simulink model "SMO_atan2_disc_model"  (R2024b)
settings: Solver=ode23  StartTime=0.0  StopTime=0.2  FixedStep=2e-7  RelTol=1e-3
InitFcn:
  | pn = 4;
  | Ld = 8.5e-3;
  | Lq = 8.5e-3;
  | Ls = Ld;
  | R = 2.875;
  | phi = 0.175;
  | J = 0.001;
  | B = 0.000;
undefined symbols (not defined in the file or in its folder): DiscIntNeverNeededParam
libraries: spsGroundLib x1, spsUniversalBridgeLib x1, spsPermanentMagnetSynchronousMachineLib x1, spsSVPWMGenerator2LevelLib x1, spsThreePhaseVIMeasurementLib x1, spsDCVoltageSourceLib x1, sps_lib x1

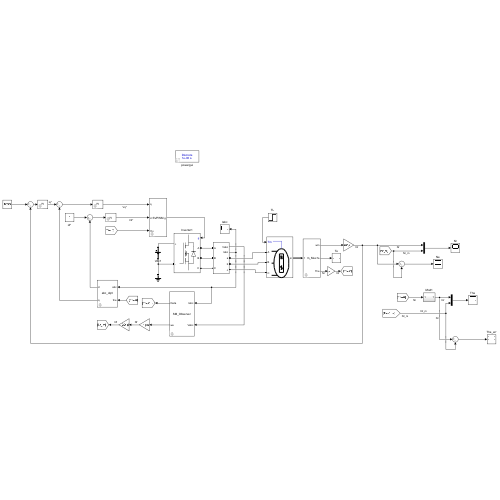
[thumbnail: Simulink's stored preview of the top-level diagram]
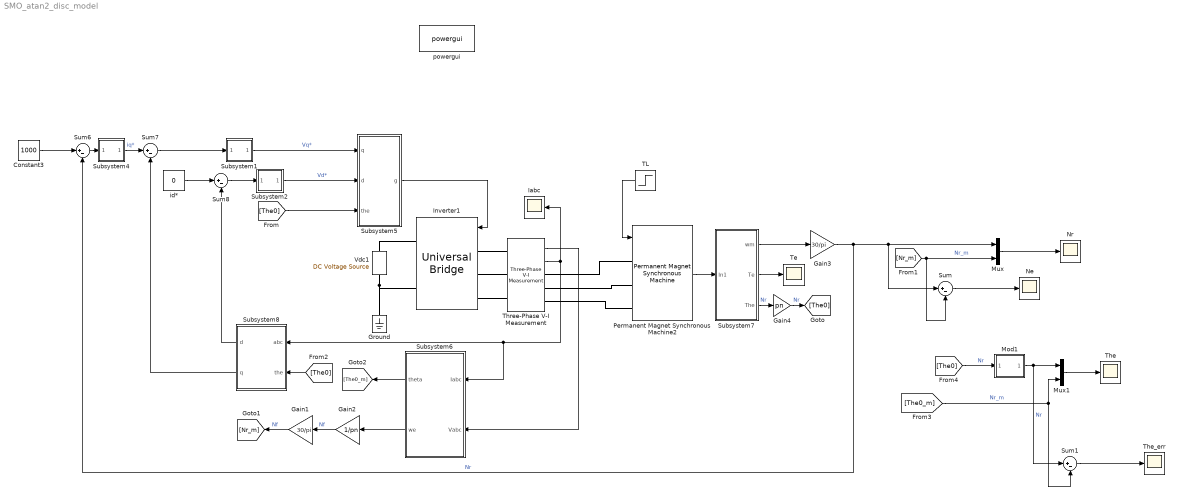
== system SMO_atan2_disc_model ==
  Constant3 : Constant  Value=1000
  Gain1 : Gain  Gain=30/pi
  Gain2 : Gain  Gain=1/pn
  Gain3 : Gain  Gain=30/pi
  Gain4 : Gain  Gain=pn
  Ground : spsGroundLib/Ground  LConnTagsString=a
  Iabc : Scope
  Inverter1 : spsUniversalBridgeLib/Universal Bridge  Arms=3  SnubberResistance=1e5  SnubberCapacitance=inf  Device=MOSFET / Diodes  Ron=1e-3  Lon=0  ForwardVoltages="[  0  0  ]"  ForwardVoltage=0  GTOparameters=[ 10e-6 , 20e-6 ]  IGBTparameters=[ 1e-6 , 2e-6 ]  Measurements=None  Measurements_2=None  converterType=Rectifier
  Mod1 : Subsystem
  Mux : Mux  Inputs=2
  Mux1 : Mux  Inputs=2
  Ne : Scope
  Nr : Scope
  Permanent Magnet Synchronous Machine2 : spsPermanentMagnetSynchronousMachineLib/Permanent Magnet Synchronous Machine  NbPhases=3  FluxDistribution=Sinusoidal  RotorType=Salient-pole  MechanicalLoad=Torque Tm  PresetModel=No  ShowDetailedParameters=on  MeasurementBus=off  Resistance=R  Inductance=8.5e-3  dqInductances=[Ld Lq]  La=0.000395  MachineConstant=Flux linkage established by magnets (V.s)  Flux=0.175  VoltageCst=126.966  TorqueCst=1.05  Flat=120  Mechanical=[J B pn 0]  PolePairs=2  InitialConditions=[0,0, 0,0]  InitialConditions5ph=[0 0 0 0 0 0]  RefAngle=Aligned with phase A axis (original Park)  IterativeDiscreteModel=Trapezoidal non iterative  TsBlock=-1  TsPowergui=0
  Subsystem1 : Subsystem  mask{Ki=2000*R, Kp=2000*Lq, int_limit=[-161,161], out_limit=[-161,161], Ts=1/(10e3)}
      mask prompts: Ki "Ki : Integral"; Kp "Kp : Propotional"; int_limit "integral limit : [min, max]"; out_limit "output limit : [min, max]"; Ts "Ts : sample time"
  Subsystem2 : Subsystem  mask{Ki=2000*R, Kp=2000*Ld, int_limit=[-161,161], out_limit=[-161,161], Ts=1/(10e3)}
      mask prompts: Ki "Ki : Integral"; Kp "Kp : Propotional"; int_limit "integral limit : [min, max]"; out_limit "output limit : [min, max]"; Ts "Ts : sample time"
  Subsystem4 : Subsystem  mask{Ki=25, Kp=0.15, int_limit=[-21,21], out_limit=[-21,21], Ts=1/(5e3)}
      mask prompts: Ki "Ki : Integral"; Kp "Kp : Propotional"; int_limit "integral limit : [min, max]"; out_limit "output limit : [min, max]"; Ts "Ts : sample time"
  Subsystem5 : Subsystem  mask{Vdc=311}
  Subsystem6 : Subsystem  mask{Ts=1/(10e3), wc=5}
      mask prompts: Ts "Ts : sample time"; wc "wc : cross frequency (rad/s)"
  Subsystem7 : Subsystem
  Subsystem8 : Subsystem
  Sum{,1,6..8} (5 alike) : Sum  Inputs=|+-
  TL : Step  Time=0.1  After=10  SampleTime=0
  Te : Scope
  The : Scope
  The_err : Scope
  Three-Phase V-I Measurement : spsThreePhaseVIMeasurementLib/Three-Phase V-I Measurement  VoltageMeasurement=phase-to-ground  SetLabelV=off  LabelV=Vabc  Vpu=off  VpuLL=off  CurrentMeasurement=yes  SetLabelI=off  LabelI=Iabc  Ipu=off  Pbase=100e6  Vbase=500e3  OutputType=Complex  PhasorSimulation=off  PSBequivalent=0
  Vdc1 : spsDCVoltageSourceLib/DC Voltage Source  Amplitude=311  Measurements=None
  id* : Constant  Value=0
  powergui : sps_lib/powergui  Priority=1  SimulationMode=Discrete  SampleTime=10e-7  frequency=60  Iterations=50  frequencyindice=0  Pbase=100e6  ErrMax=1e-4  UnitsV=kV  UnitsW=MW  buscounter=0  FunctionMessages=off  echomessages=off  EnableUseOfTLC=off  CurrentSourceSwitches=off  DisableSnubberDevices=off  DisableRonSwitches=off  DisableVfSwitches=off  DisplayEquations=off  AutomaticDiscreteSolvers=off  SolverType=Tustin/Backward Euler (TBE)  Interpol=off  ExternalGateDelay=off  methode=off  Ts=100  x0status=blocks  SPID=on  SwTol=0  HookPort=off  NonlinearTolerance=1e-4  nMaxIteration=100  ContinueOnMaxIteration=off  RestoreLinks=warning  ResistiveCurrentMeasurement=off  Frange=[0:2:500]  Ylog=off  Xlog=on  ShowGrid=off  save=off  variable=ZData  structure=0  ZoomFFT=off  StartTime=0.0  cycles=1  DisplayStyle=1  fundamental=60  FreqAxis=off  MaxFrequency=1000  frequencyindicesteady=1  RmsSteady=1  display=off
  wires:
  Three-Phase V-I Measurement/2 -> Subsystem8/1(abc), Subsystem6/1(Iabc), Iabc/1
  Sum7/1 -> Subsystem1/1(Input)
  Sum6/1 -> Subsystem4/1(Input)
  Three-Phase V-I Measurement/1 -> Subsystem6/2(Vabc)
  Subsystem4/1(output) -> Sum7/1  "iq*"
  Constant3/1 -> Sum6/1
  Subsystem5/1(g) -> Inverter1/1
  Subsystem7/1(wm) -> Gain3/1
  id*/1 -> Sum8/1
  Subsystem1/1(output) -> Subsystem5/1(q)  "Vq*"
  Sum8/1 -> Subsystem2/1(Input)
  Subsystem2/1(output) -> Subsystem5/2(d)  "Vd*"
  Subsystem8/1(d) -> Sum8/2
  Subsystem8/2(q) -> Sum7/2
  Subsystem7/2(Te) -> Te/1
  [The0] -> Subsystem5/3(the)
  Gain2/1 -> Gain1/1  "Nf"
  Subsystem6/2(we) -> Gain2/1
  Gain3/1 -> Sum6/2, Mux/1, Sum/1  "Nr"
  Mux/1 -> Nr/1
  Sum/1 -> Ne/1
  Subsystem7/3(The) -> Gain4/1  "Nr"
  TL/1 -> Permanent Magnet Synchronous Machine2/1
  Permanent Magnet Synchronous Machine2/1 -> Subsystem7/1(In1)
  [The0] -> Subsystem8/2(the)
  Gain4/1 -> [The0]  "Nr"
  Gain1/1 -> [Nr_m]  "Nf"
  [Nr_m] -> Sum/2, Mux/2  "Nr_m"
  Subsystem6/1(theta) -> [The0_m]
  [The0] -> Mod1/1(In1)  "Nr"
  Mux1/1 -> The/1
  [The0_m] -> Mux1/2, Sum1/2  "Nr_m"
  Mod1/1(Out1) -> Sum1/1, Mux1/1  "Nr"
  Sum1/1 -> The_err/1
  connections:
  Vdc1/LConn1 -- Inverter1/RConn2 -- Ground/LConn1
  Three-Phase V-I Measurement/LConn3 -- Inverter1/LConn3
  Vdc1/RConn1 -- Inverter1/RConn1
  Three-Phase V-I Measurement/LConn2 -- Inverter1/LConn2
  Three-Phase V-I Measurement/LConn1 -- Inverter1/LConn1
  Three-Phase V-I Measurement/RConn3 -- Permanent Magnet Synchronous Machine2/LConn3
  Three-Phase V-I Measurement/RConn2 -- Permanent Magnet Synchronous Machine2/LConn2
  Three-Phase V-I Measurement/RConn1 -- Permanent Magnet Synchronous Machine2/LConn1

== system SMO_atan2_disc_model/Mod1 ==
  In1 : Inport
  Constant1 : Constant  Value=2*pi
  Math Function : Math  Operator=mod  SignedPower=on
  Out1 : Outport
  wires:
  In1/1 -> Math Function/1
  Math Function/1 -> Out1/1
  Constant1/1 -> Math Function/2

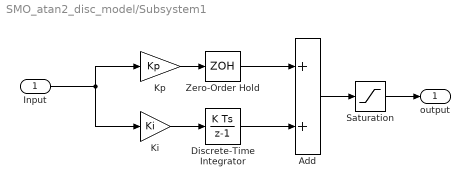
== system SMO_atan2_disc_model/Subsystem1 ==
  Input : Inport
  Add : Sum
  Discrete-Time Integrator : DiscreteIntegrator  SampleTime=Ts  LimitOutput=on  UpperSaturationLimit=int_limit(2)  LowerSaturationLimit=int_limit(1)  ICPrevOutput=DiscIntNeverNeededParam  ICPrevScaledInput=DiscIntNeverNeededParam
  Ki : Gain  Gain=Ki
  Kp : Gain  Gain=Kp
  Saturation : Saturate  UpperLimit=out_limit(2)  LowerLimit=out_limit(1)
  Zero-Order Hold : ZeroOrderHold  SampleTime=-1
  output : Outport
  wires:
  Input/1 -> Ki/1, Kp/1
  Ki/1 -> Discrete-Time Integrator/1
  Discrete-Time Integrator/1 -> Add/2
  Add/1 -> Saturation/1
  Saturation/1 -> output/1
  Kp/1 -> Zero-Order Hold/1
  Zero-Order Hold/1 -> Add/1

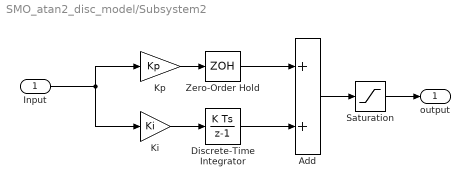
== system SMO_atan2_disc_model/Subsystem2 ==
  Input : Inport
  Add : Sum
  Discrete-Time Integrator : DiscreteIntegrator  SampleTime=Ts  LimitOutput=on  UpperSaturationLimit=int_limit(2)  LowerSaturationLimit=int_limit(1)  ICPrevOutput=DiscIntNeverNeededParam  ICPrevScaledInput=DiscIntNeverNeededParam
  Ki : Gain  Gain=Ki
  Kp : Gain  Gain=Kp
  Saturation : Saturate  UpperLimit=out_limit(2)  LowerLimit=out_limit(1)
  Zero-Order Hold : ZeroOrderHold  SampleTime=-1
  output : Outport
  wires:
  Input/1 -> Ki/1, Kp/1
  Ki/1 -> Discrete-Time Integrator/1
  Discrete-Time Integrator/1 -> Add/2
  Add/1 -> Saturation/1
  Saturation/1 -> output/1
  Kp/1 -> Zero-Order Hold/1
  Zero-Order Hold/1 -> Add/1

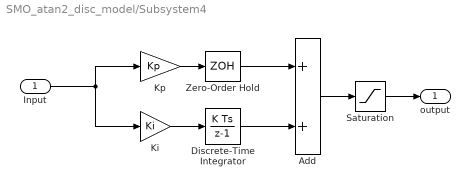
== system SMO_atan2_disc_model/Subsystem4 ==
  Input : Inport
  Add : Sum
  Discrete-Time Integrator : DiscreteIntegrator  SampleTime=Ts  LimitOutput=on  UpperSaturationLimit=int_limit(2)  LowerSaturationLimit=int_limit(1)  ICPrevOutput=DiscIntNeverNeededParam  ICPrevScaledInput=DiscIntNeverNeededParam
  Ki : Gain  Gain=Ki
  Kp : Gain  Gain=Kp
  Saturation : Saturate  UpperLimit=out_limit(2)  LowerLimit=out_limit(1)
  Zero-Order Hold : ZeroOrderHold  SampleTime=Ts
  output : Outport
  wires:
  Input/1 -> Ki/1, Kp/1
  Ki/1 -> Discrete-Time Integrator/1
  Discrete-Time Integrator/1 -> Add/2
  Add/1 -> Saturation/1
  Saturation/1 -> output/1
  Kp/1 -> Zero-Order Hold/1
  Zero-Order Hold/1 -> Add/1

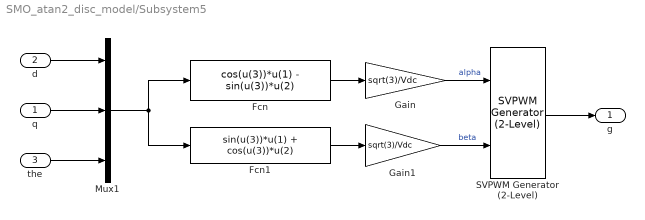
== system SMO_atan2_disc_model/Subsystem5 ==
  q : Inport
  d : Inport  Port=2
  the : Inport  Port=3
  Fcn : Fcn  Expr=cos(u(3))*u(1) - sin(u(3))*u(2)
  Fcn1 : Fcn  Expr=sin(u(3))*u(1) + cos(u(3))*u(2)
  Gain : Gain  Gain=sqrt(3)/Vdc
  Gain1 : Gain  Gain=sqrt(3)/Vdc
  Mux1 : Mux  Inputs=3
  SVPWM Generator (2-Level) : spsSVPWMGenerator2LevelLib/SVPWM Generator (2-Level)  InputType=alpha-beta components  SwitchingPattern=Pattern #1  Fc=10e3  ParUref=[0.8 -30 50]  Ts=0
  g : Outport
  wires:
  q/1 -> Mux1/2
  Fcn/1 -> Gain/1
  d/1 -> Mux1/1
  Fcn1/1 -> Gain1/1
  SVPWM Generator (2-Level)/1 -> g/1
  Mux1/1 -> Fcn/1, Fcn1/1
  the/1 -> Mux1/3
  Gain/1 -> SVPWM Generator (2-Level)/1  "alpha"
  Gain1/1 -> SVPWM Generator (2-Level)/2  "beta"

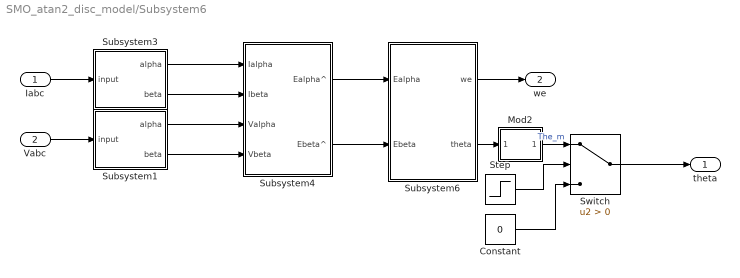
== system SMO_atan2_disc_model/Subsystem6 ==
  Iabc : Inport
  Vabc : Inport  Port=2
  Constant : Constant  Value=0
  Mod2 : Subsystem
  Step : Step  Time=0.001  SampleTime=0
  Subsystem1 : Subsystem
  Subsystem3 : Subsystem
  Subsystem4 : Subsystem
  Subsystem6 : Subsystem
  Switch : Switch  Criteria=u2 > Threshold  SaturateOnIntegerOverflow=off  InputSameDT=off
  theta : Outport
  we : Outport  Port=2
  wires:
  Subsystem4/2(Ebeta^) -> Subsystem6/2(Ebeta)
  Subsystem6/1(we) -> we/1
  Subsystem4/1(Ealpha^) -> Subsystem6/1(Ealpha)
  Iabc/1 -> Subsystem3/1(input)
  Vabc/1 -> Subsystem1/1(input)
  Subsystem3/2(beta) -> Subsystem4/2(Ibeta)
  Subsystem1/2(beta) -> Subsystem4/4(Vbeta)
  Subsystem3/1(alpha) -> Subsystem4/1(Ialpha)
  Subsystem1/1(alpha) -> Subsystem4/3(Valpha)
  Subsystem6/2(theta) -> Mod2/1(In1)
  Mod2/1(theta) -> Switch/1  "The_m"
  Switch/1 -> theta/1
  Step/1 -> Switch/2
  Constant/1 -> Switch/3

== system SMO_atan2_disc_model/Subsystem7 ==
  In1 : Inport
  Bus Selector1 : BusSelector  OutputSignals=Rotor speed wm (rad/s),Electromagnetic torque Te (N*m),Rotor angle thetam (rad)
  wm : Outport
  Te : Outport  Port=2
  The : Outport  Port=3
  wires:
  In1/1 -> Bus Selector1/1
  Bus Selector1/1 -> wm/1  "<Rotor speed wm (rad/s)>"
  Bus Selector1/2 -> Te/1  "<Electromagnetic torque Te (N*m)>"
  Bus Selector1/3 -> The/1  "<Rotor angle thetam (rad)>"

== system SMO_atan2_disc_model/Subsystem8 ==
  abc : Inport
  the : Inport  Port=2
  Subsystem : Subsystem
  Subsystem5 : Subsystem
  d : Outport
  q : Outport  Port=2
  wires:
  Subsystem/1(d) -> d/1
  the/1 -> Subsystem/3(the)
  Subsystem5/2(beta) -> Subsystem/2(beta)
  Subsystem5/1(alpha) -> Subsystem/1(alpha)
  abc/1 -> Subsystem5/1(input)
  Subsystem/2(q) -> q/1

== system SMO_atan2_disc_model/Subsystem6/Mod2 ==
  In1 : Inport
  Constant1 : Constant  Value=2*pi
  Math Function : Math  Operator=mod  SignedPower=on
  theta : Outport
  wires:
  In1/1 -> Math Function/1
  Math Function/1 -> theta/1
  Constant1/1 -> Math Function/2

== system SMO_atan2_disc_model/Subsystem6/Subsystem1 ==
  input : Inport
  Demux : Demux  Outputs=3
  Subsystem : Subsystem
  alpha : Outport
  beta : Outport  Port=2
  wires:
  input/1 -> Demux/1
  Demux/1 -> Subsystem/1(a)
  Demux/2 -> Subsystem/2(b)
  Demux/3 -> Subsystem/3(c)
  Subsystem/1(alpha) -> alpha/1
  Subsystem/2(beta) -> beta/1

== system SMO_atan2_disc_model/Subsystem6/Subsystem3 ==
  input : Inport
  Demux : Demux  Outputs=3
  Subsystem : Subsystem
  alpha : Outport
  beta : Outport  Port=2
  wires:
  input/1 -> Demux/1
  Demux/1 -> Subsystem/1(a)
  Demux/2 -> Subsystem/2(b)
  Demux/3 -> Subsystem/3(c)
  Subsystem/1(alpha) -> alpha/1
  Subsystem/2(beta) -> beta/1

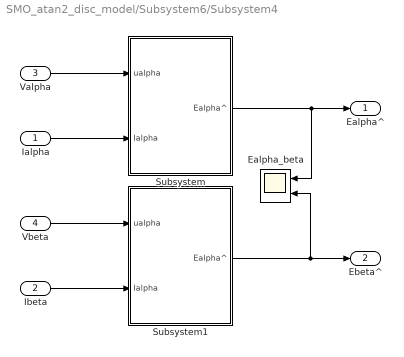
== system SMO_atan2_disc_model/Subsystem6/Subsystem4 ==
  Ialpha : Inport
  Ibeta : Inport  Port=2
  Valpha : Inport  Port=3
  Vbeta : Inport  Port=4
  Ealpha_beta : Scope  NumInputPorts=2
  Subsystem : Subsystem
  Subsystem1 : Subsystem
  Ealpha^ : Outport
  Ebeta^ : Outport  Port=2
  wires:
  Subsystem1/1(Ealpha^) -> Ebeta^/1, Ealpha_beta/2
  Valpha/1 -> Subsystem/1(ualpha)
  Ialpha/1 -> Subsystem/2(Ialpha)
  Vbeta/1 -> Subsystem1/1(ualpha)
  Ibeta/1 -> Subsystem1/2(Ialpha)
  Subsystem/1(Ealpha^) -> Ealpha^/1, Ealpha_beta/1

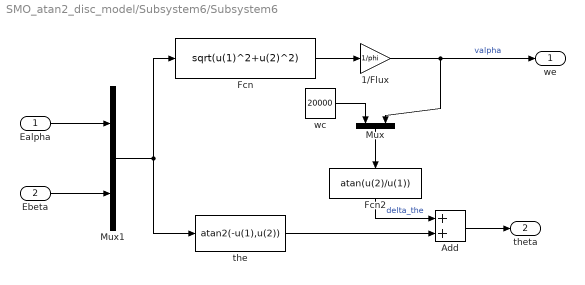
== system SMO_atan2_disc_model/Subsystem6/Subsystem6 ==
  Ealpha : Inport
  Ebeta : Inport  Port=2
  1/Flux : Gain  Gain=1/phi
  Add : Sum
  Fcn : Fcn  Expr=sqrt(u(1)^2+u(2)^2)
  Fcn2 : Fcn  Expr=atan(u(2)/u(1))
  Mux : Mux  Inputs=2
  Mux1 : Mux  Inputs=2
  the : Fcn  Expr=atan2(-u(1),u(2))
  wc : Constant  Value=20000
  we : Outport
  theta : Outport  Port=2
  wires:
  Mux1/1 -> Fcn/1, the/1
  Ebeta/1 -> Mux1/2
  Ealpha/1 -> Mux1/1
  Fcn/1 -> 1/Flux/1
  Mux/1 -> Fcn2/1
  wc/1 -> Mux/1
  Fcn2/1 -> Add/1  "delta_the"
  the/1 -> Add/2
  Add/1 -> theta/1
  1/Flux/1 -> we/1, Mux/2  "valpha"

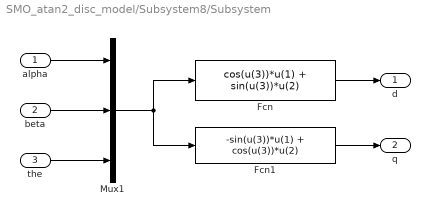
== system SMO_atan2_disc_model/Subsystem8/Subsystem ==
  alpha : Inport
  beta : Inport  Port=2
  the : Inport  Port=3
  Fcn : Fcn  Expr=cos(u(3))*u(1) + sin(u(3))*u(2)
  Fcn1 : Fcn  Expr=-sin(u(3))*u(1) + cos(u(3))*u(2)
  Mux1 : Mux  Inputs=3
  d : Outport
  q : Outport  Port=2
  wires:
  Fcn/1 -> d/1
  Mux1/1 -> Fcn/1, Fcn1/1
  the/1 -> Mux1/3
  beta/1 -> Mux1/2
  Fcn1/1 -> q/1
  alpha/1 -> Mux1/1

== system SMO_atan2_disc_model/Subsystem8/Subsystem5 ==
  input : Inport
  Demux : Demux  Outputs=3
  Subsystem : Subsystem
  alpha : Outport
  beta : Outport  Port=2
  wires:
  input/1 -> Demux/1
  Demux/1 -> Subsystem/1(a)
  Demux/2 -> Subsystem/2(b)
  Demux/3 -> Subsystem/3(c)
  Subsystem/1(alpha) -> alpha/1
  Subsystem/2(beta) -> beta/1

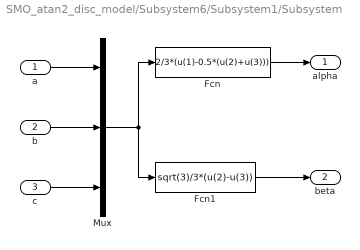
== system SMO_atan2_disc_model/Subsystem6/Subsystem1/Subsystem ==
  a : Inport
  b : Inport  Port=2
  c : Inport  Port=3
  Fcn : Fcn  Expr=2/3*(u(1)-0.5*(u(2)+u(3)))
  Fcn1 : Fcn  Expr=sqrt(3)/3*(u(2)-u(3))
  Mux : Mux  Inputs=3
  alpha : Outport
  beta : Outport  Port=2
  wires:
  a/1 -> Mux/1
  b/1 -> Mux/2
  c/1 -> Mux/3
  Mux/1 -> Fcn/1, Fcn1/1
  Fcn/1 -> alpha/1
  Fcn1/1 -> beta/1

== system SMO_atan2_disc_model/Subsystem6/Subsystem3/Subsystem ==
  a : Inport
  b : Inport  Port=2
  c : Inport  Port=3
  Fcn : Fcn  Expr=2/3*(u(1)-0.5*(u(2)+u(3)))
  Fcn1 : Fcn  Expr=sqrt(3)/3*(u(2)-u(3))
  Mux : Mux  Inputs=3
  alpha : Outport
  beta : Outport  Port=2
  wires:
  a/1 -> Mux/1
  b/1 -> Mux/2
  c/1 -> Mux/3
  Mux/1 -> Fcn/1, Fcn1/1
  Fcn/1 -> alpha/1
  Fcn1/1 -> beta/1

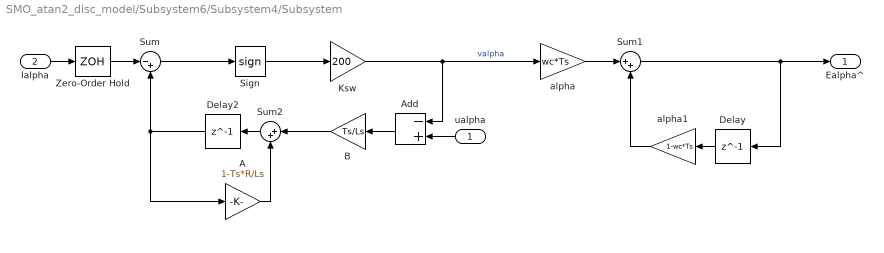
== system SMO_atan2_disc_model/Subsystem6/Subsystem4/Subsystem ==
  ualpha : Inport
  Ialpha : Inport  Port=2
  A : Gain  Gain=1-Ts*R/Ls
  Add : Sum  Inputs=-+
  B : Gain  Gain=Ts/Ls
  Delay : Delay  DelayLength=1
  Delay2 : Delay  DelayLength=1
  Ksw : Gain  Gain=200
  Sign : Signum
  Sum : Sum  Inputs=|-+
  Sum1 : Sum  Inputs=|++
  Sum2 : Sum  Inputs=|++
  Zero-Order Hold : ZeroOrderHold  SampleTime=Ts
  alpha : Gain  Gain=wc*Ts
  alpha1 : Gain  Gain=1-wc*Ts
  Ealpha^ : Outport
  wires:
  Ksw/1 -> alpha/1, Add/1  "valpha"
  Sum/1 -> Sign/1
  Sign/1 -> Ksw/1
  ualpha/1 -> Add/2
  Add/1 -> B/1
  B/1 -> Sum2/1
  Ialpha/1 -> Zero-Order Hold/1
  Zero-Order Hold/1 -> Sum/1
  A/1 -> Sum2/2
  Delay2/1 -> A/1, Sum/2
  Sum2/1 -> Delay2/1
  Delay/1 -> alpha1/1
  alpha/1 -> Sum1/1
  Sum1/1 -> Delay/1, Ealpha^/1
  alpha1/1 -> Sum1/2

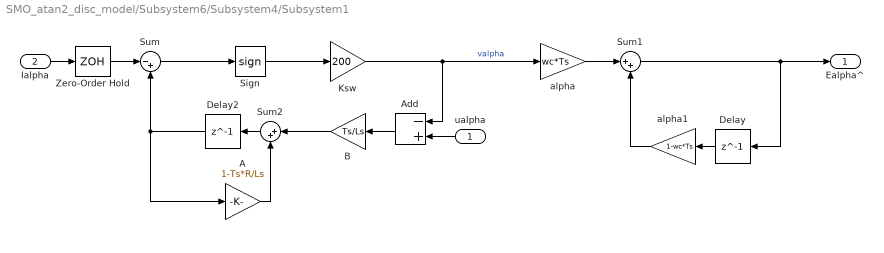
== system SMO_atan2_disc_model/Subsystem6/Subsystem4/Subsystem1 ==
  ualpha : Inport
  Ialpha : Inport  Port=2
  A : Gain  Gain=1-Ts*R/Ls
  Add : Sum  Inputs=-+
  B : Gain  Gain=Ts/Ls
  Delay : Delay  DelayLength=1
  Delay2 : Delay  DelayLength=1
  Ksw : Gain  Gain=200
  Sign : Signum
  Sum : Sum  Inputs=|-+
  Sum1 : Sum  Inputs=|++
  Sum2 : Sum  Inputs=|++
  Zero-Order Hold : ZeroOrderHold  SampleTime=Ts
  alpha : Gain  Gain=wc*Ts
  alpha1 : Gain  Gain=1-wc*Ts
  Ealpha^ : Outport
  wires:
  Ksw/1 -> alpha/1, Add/1  "valpha"
  Sum/1 -> Sign/1
  Sign/1 -> Ksw/1
  ualpha/1 -> Add/2
  Add/1 -> B/1
  B/1 -> Sum2/1
  Ialpha/1 -> Zero-Order Hold/1
  Zero-Order Hold/1 -> Sum/1
  A/1 -> Sum2/2
  Delay2/1 -> A/1, Sum/2
  Sum2/1 -> Delay2/1
  Delay/1 -> alpha1/1
  alpha/1 -> Sum1/1
  Sum1/1 -> Delay/1, Ealpha^/1
  alpha1/1 -> Sum1/2

== system SMO_atan2_disc_model/Subsystem8/Subsystem5/Subsystem ==
  a : Inport
  b : Inport  Port=2
  c : Inport  Port=3
  Fcn : Fcn  Expr=2/3*(u(1)-0.5*(u(2)+u(3)))
  Fcn1 : Fcn  Expr=sqrt(3)/3*(u(2)-u(3))
  Mux : Mux  Inputs=3
  alpha : Outport
  beta : Outport  Port=2
  wires:
  a/1 -> Mux/1
  b/1 -> Mux/2
  c/1 -> Mux/3
  Mux/1 -> Fcn/1, Fcn1/1
  Fcn/1 -> alpha/1
  Fcn1/1 -> beta/1
